simulink model "ModelOV"  (Simulink 7.4)
settings: Solver=ode45  StartTime=0.0  StopTime=250  RelTol=1e-5
settings Model: Creator=Lluís  LastModifiedBy=Lluís

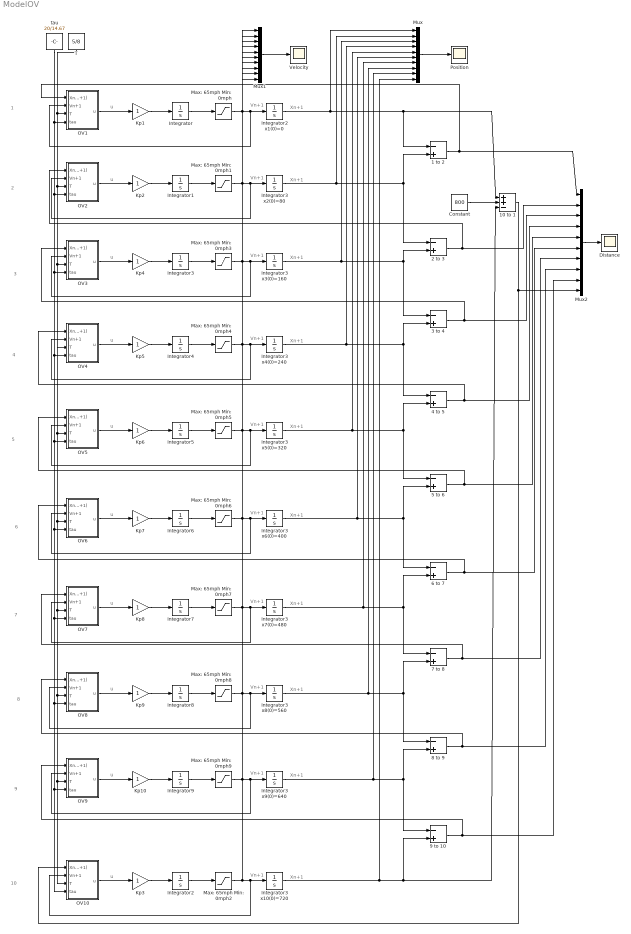
== system ModelOV ==
  note: u
  note: Vn+1
  note: Xn+1
  note: u
  note: Vn+1
  note: Xn+1
  note: 1
  note: 2
  note: u
  note: Vn+1
  note: Xn+1
  note: 10
  note: u
  note: Vn+1
  note: Xn+1
  note: 3
  note: u
  note: Vn+1
  note: Xn+1
  note: 4
  note: u
  note: Vn+1
  note: Xn+1
  note: 5
  note: u
  note: Vn+1
  note: Xn+1
  note: 6
  note: u
  note: Vn+1
  note: Xn+1
  note: 7
  note: u
  note: Vn+1
  note: Xn+1
  note: 8
  note: u
  note: Vn+1
  note: Xn+1
  note: 9
  1 to 2 : Sum  Inputs=-+  OutDataType=fixdt(1, 16)  OutScaling=2^-10
  10 to 1 : Sum  Inputs=++-  OutDataType=fixdt(1, 16)  OutScaling=2^-10
  2 to 3 : Sum  Inputs=-+  OutDataType=fixdt(1, 16)  OutScaling=2^-10
  3 to 4 : Sum  Inputs=-+  OutDataType=fixdt(1, 16)  OutScaling=2^-10
  4 to 5 : Sum  Inputs=-+  OutDataType=fixdt(1, 16)  OutScaling=2^-10
  5 to 6 : Sum  Inputs=-+  OutDataType=fixdt(1, 16)  OutScaling=2^-10
  6 to 7 : Sum  Inputs=-+  OutDataType=fixdt(1, 16)  OutScaling=2^-10
  7 to 8 : Sum  Inputs=-+  OutDataType=fixdt(1, 16)  OutScaling=2^-10
  8 to 9 : Sum  Inputs=-+  OutDataType=fixdt(1, 16)  OutScaling=2^-10
  9 to 10 : Sum  Inputs=-+  OutDataType=fixdt(1, 16)  OutScaling=2^-10
  Constant : Constant  Value=800  OutDataType=fixdt(1, 16)  OutScaling=2^0
  Distance : Scope
      settings: SaveName=ScopeData3
  Integrator : Integrator  InitialCondition=22
  Integrator{1..2,4,6,8} (5 alike) : Integrator  InitialCondition=66
  Integrator2 x1(0)=0 : Integrator
  Integrator3 : Integrator  InitialCondition=44
  Integrator3 x10(0)=720 : Integrator  InitialCondition=720
  Integrator3 x2(0)=80 : Integrator  InitialCondition=80
  Integrator3 x3(0)=160 : Integrator  InitialCondition=160
  Integrator3 x4(0)=240 : Integrator  InitialCondition=240
  Integrator3 x5(0)=320 : Integrator  InitialCondition=320
  Integrator3 x6(0)=400 : Integrator  InitialCondition=400
  Integrator3 x7(0)=480 : Integrator  InitialCondition=480
  Integrator3 x8(0)=560 : Integrator  InitialCondition=560
  Integrator3 x9(0)=640 : Integrator  InitialCondition=640
  Integrator5 : Integrator  InitialCondition=22
  Integrator7 : Integrator  InitialCondition=44
  Integrator9 : Integrator  InitialCondition=22
  Kp{1..10} (10 alike) : Gain  ParameterDataType=fixdt(1, 16)  ParameterScaling=2^0  OutDataType=fixdt(1, 16)  OutScaling=2^0
  Max: 65mph Min: 0mph{,1..9} (10 alike) : Saturate  UpperLimit=95.33  LowerLimit=0  OutDataType=fixdt(1, 16)  OutScaling=2^0
  Mux : Mux  Inputs=10
  Mux1 : Mux  Inputs=10
  Mux2 : Mux  Inputs=10
  OV1 : Subsystem
  OV10 : Subsystem
  OV2 : Subsystem
  OV3 : Subsystem
  OV4 : Subsystem
  OV5 : Subsystem
  OV6 : Subsystem
  OV7 : Subsystem
  OV8 : Subsystem
  OV9 : Subsystem
  Position : Scope
      settings: SaveName=pos
  T : Constant  Value=5/8  OutDataType=fixdt(1, 16)  OutScaling=2^0
  Velocity : Scope
      settings: SaveName=speed
  tau : Constant  Value=20/14.67  OutDataType=fixdt(1, 16)  OutScaling=2^0
  wires:
  1 to 2/1 -> OV1/1(Xn-(Xn+1)), Mux2/1
  Max: 65mph Min: 0mph/1 -> Integrator2 x1(0)=0/1, OV1/2(Vn+1), Mux1/1
  Kp1/1 -> Integrator/1
  OV1/1(u) -> Kp1/1
  Integrator/1 -> Max: 65mph Min: 0mph/1
  Integrator2 x1(0)=0/1 -> 1 to 2/1, 10 to 1/1, Mux/1
  Max: 65mph Min: 0mph1/1 -> Integrator3 x2(0)=80/1, OV2/2(Vn+1), Mux1/2
  Kp2/1 -> Integrator1/1
  Integrator1/1 -> Max: 65mph Min: 0mph1/1
  Integrator3 x2(0)=80/1 -> 1 to 2/2, 2 to 3/1, Mux/2
  Max: 65mph Min: 0mph2/1 -> Integrator3 x10(0)=720/1, OV10/2(Vn+1), Mux1/10
  Kp3/1 -> Integrator2/1
  OV10/1(u) -> Kp3/1
  Integrator2/1 -> Max: 65mph Min: 0mph2/1
  Integrator3 x10(0)=720/1 -> 10 to 1/3, 9 to 10/2, Mux/10
  2 to 3/1 -> Mux2/2, OV2/1(Xn-(Xn+1))
  Constant/1 -> 10 to 1/2
  10 to 1/1 -> Mux2/10, OV10/1(Xn-(Xn+1))
  Mux/1 -> Position/1
  Mux1/1 -> Velocity/1
  Mux2/1 -> Distance/1
  Max: 65mph Min: 0mph3/1 -> Integrator3 x3(0)=160/1, OV3/2(Vn+1), Mux1/3
  Kp4/1 -> Integrator3/1
  OV3/1(u) -> Kp4/1
  Integrator3/1 -> Max: 65mph Min: 0mph3/1
  Integrator3 x3(0)=160/1 -> 2 to 3/2, 3 to 4/1, Mux/3
  3 to 4/1 -> Mux2/3, OV3/1(Xn-(Xn+1))
  Max: 65mph Min: 0mph4/1 -> Integrator3 x4(0)=240/1, OV4/2(Vn+1), Mux1/4
  Kp5/1 -> Integrator4/1
  OV4/1(u) -> Kp5/1
  Integrator4/1 -> Max: 65mph Min: 0mph4/1
  Integrator3 x4(0)=240/1 -> 3 to 4/2, 4 to 5/1, Mux/4
  4 to 5/1 -> Mux2/4, OV4/1(Xn-(Xn+1))
  Max: 65mph Min: 0mph5/1 -> Integrator3 x5(0)=320/1, OV5/2(Vn+1), Mux1/5
  Kp6/1 -> Integrator5/1
  OV5/1(u) -> Kp6/1
  Integrator5/1 -> Max: 65mph Min: 0mph5/1
  Integrator3 x5(0)=320/1 -> 4 to 5/2, 5 to 6/1, Mux/5
  5 to 6/1 -> Mux2/5, OV5/1(Xn-(Xn+1))
  Max: 65mph Min: 0mph6/1 -> Integrator3 x6(0)=400/1, OV6/2(Vn+1), Mux1/6
  Kp7/1 -> Integrator6/1
  OV6/1(u) -> Kp7/1
  Integrator6/1 -> Max: 65mph Min: 0mph6/1
  Integrator3 x6(0)=400/1 -> 5 to 6/2, 6 to 7/1, Mux/6
  6 to 7/1 -> Mux2/6, OV6/1(Xn-(Xn+1))
  Max: 65mph Min: 0mph7/1 -> Integrator3 x7(0)=480/1, OV7/2(Vn+1), Mux1/7
  Kp8/1 -> Integrator7/1
  OV7/1(u) -> Kp8/1
  Integrator7/1 -> Max: 65mph Min: 0mph7/1
  Integrator3 x7(0)=480/1 -> 6 to 7/2, 7 to 8/1, Mux/7
  7 to 8/1 -> Mux2/7, OV7/1(Xn-(Xn+1))
  Max: 65mph Min: 0mph8/1 -> Integrator3 x8(0)=560/1, OV8/2(Vn+1), Mux1/8
  Kp9/1 -> Integrator8/1
  OV8/1(u) -> Kp9/1
  Integrator8/1 -> Max: 65mph Min: 0mph8/1
  Integrator3 x8(0)=560/1 -> 7 to 8/2, 8 to 9/1, Mux/8
  8 to 9/1 -> Mux2/8, OV8/1(Xn-(Xn+1))
  Max: 65mph Min: 0mph9/1 -> Integrator3 x9(0)=640/1, OV9/2(Vn+1), Mux1/9
  Kp10/1 -> Integrator9/1
  OV9/1(u) -> Kp10/1
  Integrator9/1 -> Max: 65mph Min: 0mph9/1
  Integrator3 x9(0)=640/1 -> 8 to 9/2, 9 to 10/1, Mux/9
  9 to 10/1 -> Mux2/9, OV9/1(Xn-(Xn+1))
  T/1 -> OV3/3(T), OV4/3(T), OV5/3(T), OV6/3(T), OV7/3(T), OV8/3(T), OV9/3(T), OV10/3(T), OV2/3(T), OV1/3(T)
  tau/1 -> OV1/4(tau), OV3/4(tau), OV4/4(tau), OV5/4(tau), OV6/4(tau), OV7/4(tau), OV8/4(tau), OV9/4(tau), OV10/4(tau), OV2/4(tau)
  OV2/1(u) -> Kp2/1

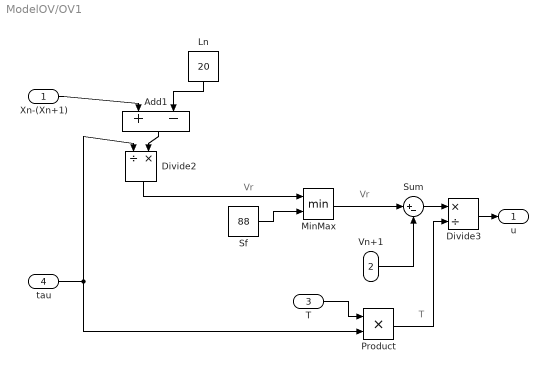
== system ModelOV/OV1 ==
  note: Vr
  note: Vr
  note: T
  Xn-(Xn+1) : Inport
  Vn+1 : Inport  Port=2
  T : Inport  Port=3  OutDataType=fixdt(1, 16)  OutScaling=2^0
  tau : Inport  Port=4  OutDataType=fixdt(1, 16)  OutScaling=2^0
  Add1 : Sum  Inputs=+-  OutDataType=fixdt(1, 16)  OutScaling=2^-10
  Divide2 : Product  Inputs=/*  OutDataType=fixdt(1, 16)  OutScaling=2^-10
  Divide3 : Product  Inputs=*/  OutDataType=fixdt(1, 16)  OutScaling=2^-10
  Ln : Constant  Value=20  OutDataType=fixdt(1, 16)  OutScaling=2^0
  MinMax : MinMax  Inputs=2  OutDataType=fixdt(1, 16)  OutScaling=2^0
  Product : Product  OutDataType=fixdt(1, 16)  OutScaling=2^0  RndMeth=Zero
  Sf : Constant  Value=88  OutDataType=fixdt(1, 16)  OutScaling=2^0
  Sum : Sum  Inputs=|+-  OutDataType=fixdt(1, 16)  OutScaling=2^0
  u : Outport
  wires:
  tau/1 -> Divide2/1, Product/2
  Ln/1 -> Add1/2
  Add1/1 -> Divide2/2
  Divide2/1 -> MinMax/1
  Xn-(Xn+1)/1 -> Add1/1
  Vn+1/1 -> Sum/2
  Sf/1 -> MinMax/2
  MinMax/1 -> Sum/1
  Sum/1 -> Divide3/1
  Product/1 -> Divide3/2
  Divide3/1 -> u/1
  T/1 -> Product/1

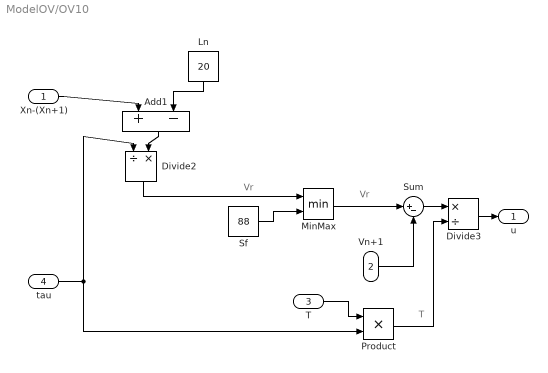
== system ModelOV/OV10 ==
  note: Vr
  note: Vr
  note: T
  Xn-(Xn+1) : Inport
  Vn+1 : Inport  Port=2
  T : Inport  Port=3  OutDataType=fixdt(1, 16)  OutScaling=2^0
  tau : Inport  Port=4  OutDataType=fixdt(1, 16)  OutScaling=2^0
  Add1 : Sum  Inputs=+-  OutDataType=fixdt(1, 16)  OutScaling=2^-10
  Divide2 : Product  Inputs=/*  OutDataType=fixdt(1, 16)  OutScaling=2^-10
  Divide3 : Product  Inputs=*/  OutDataType=fixdt(1, 16)  OutScaling=2^-10
  Ln : Constant  Value=20  OutDataType=fixdt(1, 16)  OutScaling=2^0
  MinMax : MinMax  Inputs=2  OutDataType=fixdt(1, 16)  OutScaling=2^0
  Product : Product  OutDataType=fixdt(1, 16)  OutScaling=2^0  RndMeth=Zero
  Sf : Constant  Value=88  OutDataType=fixdt(1, 16)  OutScaling=2^0
  Sum : Sum  Inputs=|+-  OutDataType=fixdt(1, 16)  OutScaling=2^0
  u : Outport
  wires:
  tau/1 -> Divide2/1, Product/2
  Ln/1 -> Add1/2
  Add1/1 -> Divide2/2
  Divide2/1 -> MinMax/1
  Xn-(Xn+1)/1 -> Add1/1
  Vn+1/1 -> Sum/2
  Sf/1 -> MinMax/2
  MinMax/1 -> Sum/1
  Sum/1 -> Divide3/1
  Product/1 -> Divide3/2
  Divide3/1 -> u/1
  T/1 -> Product/1

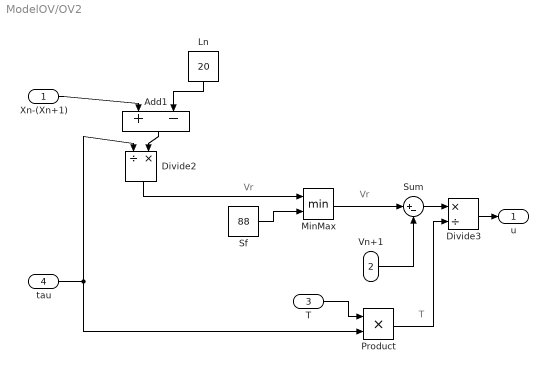
== system ModelOV/OV2 ==
  note: Vr
  note: Vr
  note: T
  Xn-(Xn+1) : Inport
  Vn+1 : Inport  Port=2
  T : Inport  Port=3  OutDataType=fixdt(1, 16)  OutScaling=2^0
  tau : Inport  Port=4  OutDataType=fixdt(1, 16)  OutScaling=2^0
  Add1 : Sum  Inputs=+-  OutDataType=fixdt(1, 16)  OutScaling=2^-10
  Divide2 : Product  Inputs=/*  OutDataType=fixdt(1, 16)  OutScaling=2^-10
  Divide3 : Product  Inputs=*/  OutDataType=fixdt(1, 16)  OutScaling=2^-10
  Ln : Constant  Value=20  OutDataType=fixdt(1, 16)  OutScaling=2^0
  MinMax : MinMax  Inputs=2  OutDataType=fixdt(1, 16)  OutScaling=2^0
  Product : Product  OutDataType=fixdt(1, 16)  OutScaling=2^0  RndMeth=Zero
  Sf : Constant  Value=88  OutDataType=fixdt(1, 16)  OutScaling=2^0
  Sum : Sum  Inputs=|+-  OutDataType=fixdt(1, 16)  OutScaling=2^0
  u : Outport
  wires:
  tau/1 -> Divide2/1, Product/2
  Ln/1 -> Add1/2
  Add1/1 -> Divide2/2
  Divide2/1 -> MinMax/1
  Xn-(Xn+1)/1 -> Add1/1
  Vn+1/1 -> Sum/2
  Sf/1 -> MinMax/2
  MinMax/1 -> Sum/1
  Sum/1 -> Divide3/1
  Product/1 -> Divide3/2
  Divide3/1 -> u/1
  T/1 -> Product/1

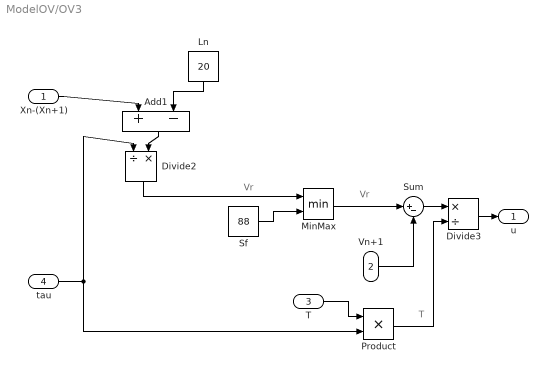
== system ModelOV/OV3 ==
  note: Vr
  note: Vr
  note: T
  Xn-(Xn+1) : Inport
  Vn+1 : Inport  Port=2
  T : Inport  Port=3  OutDataType=fixdt(1, 16)  OutScaling=2^0
  tau : Inport  Port=4  OutDataType=fixdt(1, 16)  OutScaling=2^0
  Add1 : Sum  Inputs=+-  OutDataType=fixdt(1, 16)  OutScaling=2^-10
  Divide2 : Product  Inputs=/*  OutDataType=fixdt(1, 16)  OutScaling=2^-10
  Divide3 : Product  Inputs=*/  OutDataType=fixdt(1, 16)  OutScaling=2^-10
  Ln : Constant  Value=20  OutDataType=fixdt(1, 16)  OutScaling=2^0
  MinMax : MinMax  Inputs=2  OutDataType=fixdt(1, 16)  OutScaling=2^0
  Product : Product  OutDataType=fixdt(1, 16)  OutScaling=2^0  RndMeth=Zero
  Sf : Constant  Value=88  OutDataType=fixdt(1, 16)  OutScaling=2^0
  Sum : Sum  Inputs=|+-  OutDataType=fixdt(1, 16)  OutScaling=2^0
  u : Outport
  wires:
  tau/1 -> Divide2/1, Product/2
  Ln/1 -> Add1/2
  Add1/1 -> Divide2/2
  Divide2/1 -> MinMax/1
  Xn-(Xn+1)/1 -> Add1/1
  Vn+1/1 -> Sum/2
  Sf/1 -> MinMax/2
  MinMax/1 -> Sum/1
  Sum/1 -> Divide3/1
  Product/1 -> Divide3/2
  Divide3/1 -> u/1
  T/1 -> Product/1

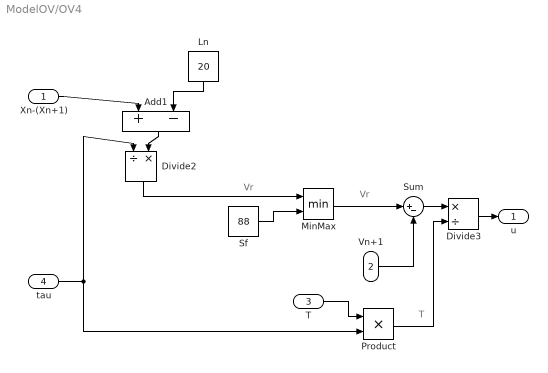
== system ModelOV/OV4 ==
  note: Vr
  note: Vr
  note: T
  Xn-(Xn+1) : Inport
  Vn+1 : Inport  Port=2
  T : Inport  Port=3  OutDataType=fixdt(1, 16)  OutScaling=2^0
  tau : Inport  Port=4  OutDataType=fixdt(1, 16)  OutScaling=2^0
  Add1 : Sum  Inputs=+-  OutDataType=fixdt(1, 16)  OutScaling=2^-10
  Divide2 : Product  Inputs=/*  OutDataType=fixdt(1, 16)  OutScaling=2^-10
  Divide3 : Product  Inputs=*/  OutDataType=fixdt(1, 16)  OutScaling=2^-10
  Ln : Constant  Value=20  OutDataType=fixdt(1, 16)  OutScaling=2^0
  MinMax : MinMax  Inputs=2  OutDataType=fixdt(1, 16)  OutScaling=2^0
  Product : Product  OutDataType=fixdt(1, 16)  OutScaling=2^0  RndMeth=Zero
  Sf : Constant  Value=88  OutDataType=fixdt(1, 16)  OutScaling=2^0
  Sum : Sum  Inputs=|+-  OutDataType=fixdt(1, 16)  OutScaling=2^0
  u : Outport
  wires:
  tau/1 -> Divide2/1, Product/2
  Ln/1 -> Add1/2
  Add1/1 -> Divide2/2
  Divide2/1 -> MinMax/1
  Xn-(Xn+1)/1 -> Add1/1
  Vn+1/1 -> Sum/2
  Sf/1 -> MinMax/2
  MinMax/1 -> Sum/1
  Sum/1 -> Divide3/1
  Product/1 -> Divide3/2
  Divide3/1 -> u/1
  T/1 -> Product/1

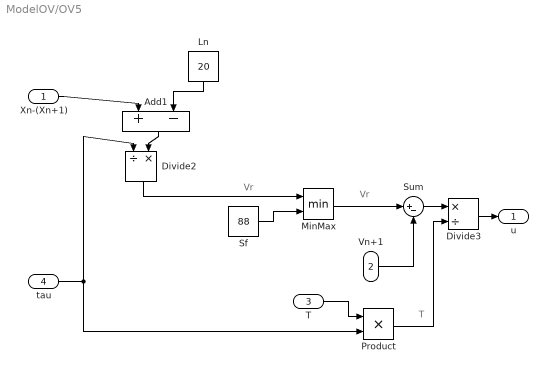
== system ModelOV/OV5 ==
  note: Vr
  note: Vr
  note: T
  Xn-(Xn+1) : Inport
  Vn+1 : Inport  Port=2
  T : Inport  Port=3  OutDataType=fixdt(1, 16)  OutScaling=2^0
  tau : Inport  Port=4  OutDataType=fixdt(1, 16)  OutScaling=2^0
  Add1 : Sum  Inputs=+-  OutDataType=fixdt(1, 16)  OutScaling=2^-10
  Divide2 : Product  Inputs=/*  OutDataType=fixdt(1, 16)  OutScaling=2^-10
  Divide3 : Product  Inputs=*/  OutDataType=fixdt(1, 16)  OutScaling=2^-10
  Ln : Constant  Value=20  OutDataType=fixdt(1, 16)  OutScaling=2^0
  MinMax : MinMax  Inputs=2  OutDataType=fixdt(1, 16)  OutScaling=2^0
  Product : Product  OutDataType=fixdt(1, 16)  OutScaling=2^0  RndMeth=Zero
  Sf : Constant  Value=88  OutDataType=fixdt(1, 16)  OutScaling=2^0
  Sum : Sum  Inputs=|+-  OutDataType=fixdt(1, 16)  OutScaling=2^0
  u : Outport
  wires:
  tau/1 -> Divide2/1, Product/2
  Ln/1 -> Add1/2
  Add1/1 -> Divide2/2
  Divide2/1 -> MinMax/1
  Xn-(Xn+1)/1 -> Add1/1
  Vn+1/1 -> Sum/2
  Sf/1 -> MinMax/2
  MinMax/1 -> Sum/1
  Sum/1 -> Divide3/1
  Product/1 -> Divide3/2
  Divide3/1 -> u/1
  T/1 -> Product/1

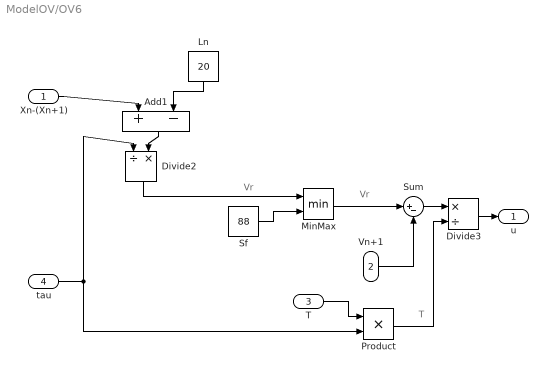
== system ModelOV/OV6 ==
  note: Vr
  note: Vr
  note: T
  Xn-(Xn+1) : Inport
  Vn+1 : Inport  Port=2
  T : Inport  Port=3  OutDataType=fixdt(1, 16)  OutScaling=2^0
  tau : Inport  Port=4  OutDataType=fixdt(1, 16)  OutScaling=2^0
  Add1 : Sum  Inputs=+-  OutDataType=fixdt(1, 16)  OutScaling=2^-10
  Divide2 : Product  Inputs=/*  OutDataType=fixdt(1, 16)  OutScaling=2^-10
  Divide3 : Product  Inputs=*/  OutDataType=fixdt(1, 16)  OutScaling=2^-10
  Ln : Constant  Value=20  OutDataType=fixdt(1, 16)  OutScaling=2^0
  MinMax : MinMax  Inputs=2  OutDataType=fixdt(1, 16)  OutScaling=2^0
  Product : Product  OutDataType=fixdt(1, 16)  OutScaling=2^0  RndMeth=Zero
  Sf : Constant  Value=88  OutDataType=fixdt(1, 16)  OutScaling=2^0
  Sum : Sum  Inputs=|+-  OutDataType=fixdt(1, 16)  OutScaling=2^0
  u : Outport
  wires:
  tau/1 -> Divide2/1, Product/2
  Ln/1 -> Add1/2
  Add1/1 -> Divide2/2
  Divide2/1 -> MinMax/1
  Xn-(Xn+1)/1 -> Add1/1
  Vn+1/1 -> Sum/2
  Sf/1 -> MinMax/2
  MinMax/1 -> Sum/1
  Sum/1 -> Divide3/1
  Product/1 -> Divide3/2
  Divide3/1 -> u/1
  T/1 -> Product/1

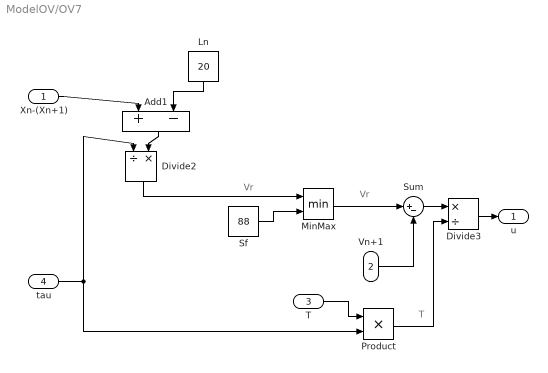
== system ModelOV/OV7 ==
  note: Vr
  note: Vr
  note: T
  Xn-(Xn+1) : Inport
  Vn+1 : Inport  Port=2
  T : Inport  Port=3  OutDataType=fixdt(1, 16)  OutScaling=2^0
  tau : Inport  Port=4  OutDataType=fixdt(1, 16)  OutScaling=2^0
  Add1 : Sum  Inputs=+-  OutDataType=fixdt(1, 16)  OutScaling=2^-10
  Divide2 : Product  Inputs=/*  OutDataType=fixdt(1, 16)  OutScaling=2^-10
  Divide3 : Product  Inputs=*/  OutDataType=fixdt(1, 16)  OutScaling=2^-10
  Ln : Constant  Value=20  OutDataType=fixdt(1, 16)  OutScaling=2^0
  MinMax : MinMax  Inputs=2  OutDataType=fixdt(1, 16)  OutScaling=2^0
  Product : Product  OutDataType=fixdt(1, 16)  OutScaling=2^0  RndMeth=Zero
  Sf : Constant  Value=88  OutDataType=fixdt(1, 16)  OutScaling=2^0
  Sum : Sum  Inputs=|+-  OutDataType=fixdt(1, 16)  OutScaling=2^0
  u : Outport
  wires:
  tau/1 -> Divide2/1, Product/2
  Ln/1 -> Add1/2
  Add1/1 -> Divide2/2
  Divide2/1 -> MinMax/1
  Xn-(Xn+1)/1 -> Add1/1
  Vn+1/1 -> Sum/2
  Sf/1 -> MinMax/2
  MinMax/1 -> Sum/1
  Sum/1 -> Divide3/1
  Product/1 -> Divide3/2
  Divide3/1 -> u/1
  T/1 -> Product/1

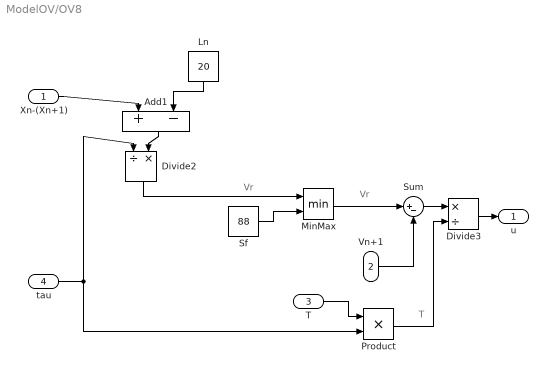
== system ModelOV/OV8 ==
  note: Vr
  note: Vr
  note: T
  Xn-(Xn+1) : Inport
  Vn+1 : Inport  Port=2
  T : Inport  Port=3  OutDataType=fixdt(1, 16)  OutScaling=2^0
  tau : Inport  Port=4  OutDataType=fixdt(1, 16)  OutScaling=2^0
  Add1 : Sum  Inputs=+-  OutDataType=fixdt(1, 16)  OutScaling=2^-10
  Divide2 : Product  Inputs=/*  OutDataType=fixdt(1, 16)  OutScaling=2^-10
  Divide3 : Product  Inputs=*/  OutDataType=fixdt(1, 16)  OutScaling=2^-10
  Ln : Constant  Value=20  OutDataType=fixdt(1, 16)  OutScaling=2^0
  MinMax : MinMax  Inputs=2  OutDataType=fixdt(1, 16)  OutScaling=2^0
  Product : Product  OutDataType=fixdt(1, 16)  OutScaling=2^0  RndMeth=Zero
  Sf : Constant  Value=88  OutDataType=fixdt(1, 16)  OutScaling=2^0
  Sum : Sum  Inputs=|+-  OutDataType=fixdt(1, 16)  OutScaling=2^0
  u : Outport
  wires:
  tau/1 -> Divide2/1, Product/2
  Ln/1 -> Add1/2
  Add1/1 -> Divide2/2
  Divide2/1 -> MinMax/1
  Xn-(Xn+1)/1 -> Add1/1
  Vn+1/1 -> Sum/2
  Sf/1 -> MinMax/2
  MinMax/1 -> Sum/1
  Sum/1 -> Divide3/1
  Product/1 -> Divide3/2
  Divide3/1 -> u/1
  T/1 -> Product/1

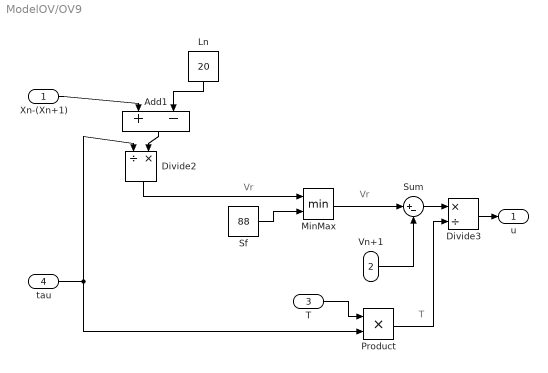
== system ModelOV/OV9 ==
  note: Vr
  note: Vr
  note: T
  Xn-(Xn+1) : Inport
  Vn+1 : Inport  Port=2
  T : Inport  Port=3  OutDataType=fixdt(1, 16)  OutScaling=2^0
  tau : Inport  Port=4  OutDataType=fixdt(1, 16)  OutScaling=2^0
  Add1 : Sum  Inputs=+-  OutDataType=fixdt(1, 16)  OutScaling=2^-10
  Divide2 : Product  Inputs=/*  OutDataType=fixdt(1, 16)  OutScaling=2^-10
  Divide3 : Product  Inputs=*/  OutDataType=fixdt(1, 16)  OutScaling=2^-10
  Ln : Constant  Value=20  OutDataType=fixdt(1, 16)  OutScaling=2^0
  MinMax : MinMax  Inputs=2  OutDataType=fixdt(1, 16)  OutScaling=2^0
  Product : Product  OutDataType=fixdt(1, 16)  OutScaling=2^0  RndMeth=Zero
  Sf : Constant  Value=88  OutDataType=fixdt(1, 16)  OutScaling=2^0
  Sum : Sum  Inputs=|+-  OutDataType=fixdt(1, 16)  OutScaling=2^0
  u : Outport
  wires:
  tau/1 -> Divide2/1, Product/2
  Ln/1 -> Add1/2
  Add1/1 -> Divide2/2
  Divide2/1 -> MinMax/1
  Xn-(Xn+1)/1 -> Add1/1
  Vn+1/1 -> Sum/2
  Sf/1 -> MinMax/2
  MinMax/1 -> Sum/1
  Sum/1 -> Divide3/1
  Product/1 -> Divide3/2
  Divide3/1 -> u/1
  T/1 -> Product/1
